simulink model "Controller"  (R2015a)
settings: Solver=ode3  SolverMode=SingleTasking  StartTime=0.0  StopTime=100  FixedStep=T_sim  RelTol=1e-3
PreLoadFcn:
  | LoadLibraries
values from neighbouring files (symbols this model uses):
  a = 10.26    [SetupComplete.m]
  A_x = 0.015    [SetupComplete.m]
  A_y = A_x    (= 0.015)    [SetupComplete.m]
  A_z = 0.16    [SetupComplete.m]
  C_d0 = 0.001193    [SetupComplete.m]
  C_x = 1.2    [SetupComplete.m]
  C_y = C_x    (= 1.2)    [SetupComplete.m]
  C_z = 2.2    [SetupComplete.m]
  CG_0 = [0,0,0.02]'    [SetupComplete.m]
  eta_23 = deg2rad(-1.42)    [Run3Copter.m]
  g = 9.81    [SetupComplete.m]
  h = 0.08    [SetupComplete.m]
  h_M = 0.064    [SetupComplete.m]
  I_BAC_0 = [ Ix,0,Ixz;0,Iy,0;Ixz,0,Iz]    [SetupComplete.m]
  Initial_Omegas = [1;1;1]*Omega_hover    [Run3Copter.m]
  l = 0.3450    (= 0.345)    [NDI_components.m]    (also in SetupComplete.m; robust_controller.m)
  l_arm = 0.264    [SetupComplete.m]
  m = 3.51    [SetupComplete.m]
  m_0 = 2.61    [SetupComplete.m]
  m_M = 0.300    (= 0.3)    [SetupComplete.m]
  R = 0.1778    [SetupComplete.m]    (also in robust_controller.m = eye(4))
  rho = 1.15    [SetupComplete.m]
  sigma = b*c/(pi*R)    (= 0.107416159567)    [SetupComplete.m]
  theta_0 = 0.38397    [SetupComplete.m]
  theta_1 = -0.2967    [SetupComplete.m]
  v_i0 = sqrt( 1/3*m*g/(2*rho*pi*R^2)  )    [SetupComplete.m]
undefined symbols (not defined in the file or in its folder): DOWN_0, EAST_0, Motor, NORTH_0, P_0, Prop, Q_0, R_0, Throttle_Hover, U_0, V_0, v_i_adim, Vx_adim, Vz_adim, W_0
undefined symbols (not defined in the file): Initial_Torques, J_FA, J_T, Rotation_sign, Tau_motors
libraries: XXCopter x39, simulink x35, vrlib x15, simulink_extras x7, aerolib6dofsys x2, qcatlib x2, dspinverses x2
(part 10 of 10)

== matlab function Controller/P Controller/NDI+CA Controller/4DOF NDI+CA Controller/F(X) ==
  data: fx output; prev_input input
function fx = fx(prev_input)
    % Calculates f_hat(x). The expression is calculated in NDI_components
    % x_dot = f(x) + g(x,u)
    %   g(x,u) ~= g(x,u0) + jac(g(x,u), u)(u0) * (u - u0)
    %   g(x,u) ~= h(x,u0) + jac(g(x,u), u)(u0) * u
    % x_dot = f_hat(x) + jac(g(x,u), u) * u
    %   f_hat(x) = f(x) + g(x,u0) - jac(g(x,u), u)(u0) *  u0
    %   g_hat(x) = jac(g(x,u), u)(u0)
    % x_dot = f_hat(x) + g_hat(x) * u
    Ixx = I_BAC(1,1);
    Iyy = I_BAC(2,2);
    Izz = I_BAC(3,3);
    Ixz = I_BAC(1,3);
    Iyz = I_BAC(2,3);
    cx = CG(1);
    cy = CG(2);
    cz = CG(3);
    tau1_0 = prev_input(1);
    eta1_0 = prev_input(2);
    gamma1_0 = prev_input(3);
    tau2_0 = prev_input(4);
    eta2_0 = prev_input(5);
    gamma2_0 = prev_input(6);
    tau3_0 = prev_input(7);
    eta3_0 = prev_input(8);
    gamma3_0 = prev_input(9);

    % TODO Precompute sines and cosines to improve performance. Some
    % repeated terms can also be precomputed
 fx = [...
               (88.941*(6.6073e-7*mass*P^2 + 0.000032054*mass*P*R - 6.6073e-7*mass*R^2 + 0.011243*V*mass*R + 0.011243*Gx - 0.011243*Q*W*mass - 5.7814e-6*eta1_0*mass*tau1_0*cos(eta1_0)))/mass;
 (88.941*(0.011243*Gy - 0.16865*eta1_0*tau1_0*cos(eta1_0) + 7.3537e-7*P*Q*mass + 0.00003163*Q*R*mass + 0.011243*P*W*mass - 0.011243*R*U*mass - 1.7153e-7*eta1_0*mass*tau1_0*sin(eta1_0)))/mass;
                                        -(88.941*(0.000016865*mass*P^2 + 0.011243*V*mass*P + 0.000016865*mass*Q^2 - 0.011243*U*mass*Q - 0.011243*Gz + 0.16865*eta1_0*tau1_0*sin(eta1_0)))/mass;
                                                                                                                               0.010171*eta1_0*tau1_0*sin(eta1_0) - 0.87546*Q*R - 0.043603*P*Q;
                                                                                                                  0.039177*P^2 + 0.90059*P*R - 0.039177*R^2 - 0.3428*eta1_0*tau1_0*cos(eta1_0);
                                                                                                                                0.043603*Q*R - 0.12686*P*Q - 0.20367*eta1_0*tau1_0*sin(eta1_0)];

== matlab function Controller/P Controller/NDI+CA Controller/4DOF NDI+CA Controller - No massic update/F(X) ==
  data: fx output size=[4,1]; prev_input input size=[9,1]; gforce_body input size=[3,1]; omega_body input size=[3,1]; v_body input size=[3,1]
function fx = fx(prev_input, gforce_body, omega_body, v_body)
    % Calculates f_hat(x). The expression is calculated in NDI_components
    % x_dot = f(x) + g(x,u)
    %   g(x,u) ~= g(x,u0) + jac(g(x,u), u)(u0) * (u - u0)
    %   g(x,u) ~= h(x,u0) + jac(g(x,u), u)(u0) * u
    % x_dot = f_hat(x) + jac(g(x,u), u) * u
    %   f_hat(x) = f(x) + g(x,u0) - jac(g(x,u), u)(u0) *  u0
    %   g_hat(x) = jac(g(x,u), u)(u0)
    % x_dot = f_hat(x) + g_hat(x) * u
    tau1_0 = prev_input(1);
    eta1_0 = prev_input(2);
    gamma1_0 = prev_input(3);
    tau2_0 = prev_input(4);
    eta2_0 = prev_input(5);
    gamma2_0 = prev_input(6);
    tau3_0 = prev_input(7);
    eta3_0 = prev_input(8);
    gamma3_0 = prev_input(9);
    Gx =  gforce_body(1);
    Gy =  gforce_body(2);
    Gz =  gforce_body(3);
    U = v_body(1);
    V = v_body(2);
    W = v_body(3);
    P = omega_body(1);
    Q = omega_body(2);
    R = omega_body(3);

    % This matrix was precomputed in NDI_components.m
    % TODO Precompute sines and cosines to improve performance. Some
    % repeated terms can also be precomputed
    
 fx = [... 
                         - 0.0015*P^2 - 1.0*V*P - 0.0015*Q^2 + 1.0*U*Q + 0.2849*Gz - 4.2735*eta1_0*tau1_0*sin(eta1_0);
                  0.89255*eta1_0*tau1_0*cos(eta1_0) - 0.87555*Q*R - 0.043605*P*Q + 0.010171*eta1_0*tau1_0*sin(eta1_0);
     0.039179*P^2 + 0.90066*P*R - 0.039179*R^2 - 0.34281*eta1_0*tau1_0*cos(eta1_0) + 25.344*eta1_0*tau1_0*sin(eta1_0);
                     0.043605*Q*R - 0.12686*P*Q - 15.06*eta1_0*tau1_0*cos(eta1_0) - 0.20367*eta1_0*tau1_0*sin(eta1_0)];

== matlab function Controller/P Controller/NDI+CA Controller/4DOF NDI+CA Controller - No massic update/G(X) 4DOF_WPQR ==
  data: gx output size=[4,4]; prev_input input size=[9,1]
function gx = gx(prev_input)
    % Calculates f_hat(x). The expression is calculated in NDI_components
    % x_dot = f(x) + g(x,u)
    %   g(x,u) ~= g(x,u0) + jac(g(x,u), u)(u0) * (u - u0)
    %   g(x,u) ~= h(x,u0) + jac(g(x,u), u)(u0) * u
    % x_dot = f_hat(x) + jac(g(x,u), u) * u
    %   f_hat(x) = f(x) + g(x,u0) - jac(g(x,u), u)(u0) *  u0
    %   g_hat(x) = jac(g(x,u), u)(u0)
    % x_dot = f_hat(x) + g_hat(x) * u
    tau1_0 = prev_input(1);
    eta1_0 = prev_input(2);
    gamma1_0 = prev_input(3);
    tau2_0 = prev_input(4);
    eta2_0 = prev_input(5);
    gamma2_0 = prev_input(6);
    tau3_0 = prev_input(7);
    eta3_0 = prev_input(8);
    gamma3_0 = prev_input(9);
    
    % This matrix was precomputed in NDI_components.m
    % TODO Precompute sines and cosines to improve performance. Some
    % repeated terms can also be precomputed
    gx = [...
                       -4.274*cos(eta1_0),                                 4.274*tau1_0*sin(eta1_0), -4.274,  -4.274;
 0.01017*cos(eta1_0) - 0.8926*sin(eta1_0), - 0.8926*tau1_0*cos(eta1_0) - 0.01017*tau1_0*sin(eta1_0), -28.02,    28.0;
   25.34*cos(eta1_0) + 0.3428*sin(eta1_0),     0.3428*tau1_0*cos(eta1_0) - 25.34*tau1_0*sin(eta1_0), -12.67,  -12.67;
   15.06*sin(eta1_0) - 0.2037*cos(eta1_0),     15.06*tau1_0*cos(eta1_0) + 0.2037*tau1_0*sin(eta1_0), 0.8549, -0.4475];


 
    
    
    
    
%  0.038016*cos(eta1_0) + 0.00051422*sin(eta1_0), 0.00051422*tau1_0*cos(eta1_0) - 0.038016*tau1_0*sin(eta1_0),    -4.2737*tau1_0, -0.019008,    -4.2737*tau2_0, -0.00051422*tau2_0, -0.019008,   -4.2737*tau3_0, -0.00051422*tau3_0;
%   4.2748*sin(eta1_0) - 0.000015257*cos(eta1_0),  4.2748*tau1_0*cos(eta1_0) + 0.000015257*tau1_0*sin(eta1_0), 0.00065622*tau1_0,  0.042029, 0.00032056*tau2_0,      4.2732*tau2_0, -0.041999, -0.001633*tau3_0,      4.2732*tau3_0;
%                            -4.2735*cos(eta1_0),                                   4.2735*tau1_0*sin(eta1_0),                 0,   -4.2735,                 0,                  0,   -4.2735,                0,                  0;
%     0.010171*cos(eta1_0) - 0.89255*sin(eta1_0),  - 0.89255*tau1_0*cos(eta1_0) - 0.010171*tau1_0*sin(eta1_0),   -0.43748*tau1_0,    -28.02,   -0.21371*tau2_0,     0.23535*tau2_0,    27.999,    1.0887*tau3_0,     0.23535*tau3_0;
%       25.344*cos(eta1_0) + 0.34281*sin(eta1_0),      0.34281*tau1_0*cos(eta1_0) - 25.344*tau1_0*sin(eta1_0),   -0.11019*tau1_0,   -12.672,   -0.11019*tau2_0,    -0.34281*tau2_0,   -12.672,  -0.11019*tau3_0,    -0.34281*tau3_0;
%        15.06*sin(eta1_0) - 0.20367*cos(eta1_0),       15.06*tau1_0*cos(eta1_0) + 0.20367*tau1_0*sin(eta1_0),   0.010171*tau1_0,   0.85486,     13.029*tau2_0,     -7.5251*tau2_0,  -0.44753,    -13.05*tau3_0,     -7.5251*tau3_0];

== matlab function Controller/P Controller/NDI+CA Controller/ 9DOF NDI+CA Controller - No massic update/F(X) 9DOF_UVWPQR ==
  data: fx output size=[6,1]; prev_input input size=[9,1]; gforce_body input size=[3,1]; omega_body input size=[3,1]; v_body input size=[3,1]
function fx = fx(prev_input, gforce_body, omega_body, v_body)
    % Calculates f_hat(x). The expression is calculated in NDI_components
    % x_dot = f(x) + g(x,u)
    %   g(x,u) ~= g(x,u0) + jac(g(x,u), u)(u0) * (u - u0)
    %   g(x,u) ~= h(x,u0) + jac(g(x,u), u)(u0) * u
    % x_dot = f_hat(x) + jac(g(x,u), u) * u
    %   f_hat(x) = f(x) + g(x,u0) - jac(g(x,u), u)(u0) *  u0
    %   g_hat(x) = jac(g(x,u), u)(u0)
    % x_dot = f_hat(x) + g_hat(x) * u
    tau1_0 = prev_input(1);
    eta1_0 = prev_input(2);
    gamma1_0 = prev_input(3);
    tau2_0 = prev_input(4);
    eta2_0 = prev_input(5);
    gamma2_0 = prev_input(6);
    tau3_0 = prev_input(7);
    eta3_0 = prev_input(8);
    gamma3_0 = prev_input(9);
    Gx =  gforce_body(1);
    Gy =  gforce_body(2);
    Gz =  gforce_body(3);
    U = v_body(1);
    V = v_body(2);
    W = v_body(3);
    P = omega_body(1);
    Q = omega_body(2);
    R = omega_body(3);

    % This matrix was precomputed in NDI_components.m
    % TODO Precompute sines and cosines to improve performance. Some
    % repeated terms can also be precomputed
    
 fx = [...
 5.88e-5*P^2 + 0.00285*P*R - 5.88e-5*R^2 + 1.0*V*R + 0.285*Gx - 1.0*Q*W + 4.27*gamma1_0*tau1_0*cos(gamma1_0) + 5.14e-4*gamma2_0*tau2_0*cos(gamma2_0) + 5.14e-4*gamma3_0*tau3_0*cos(gamma3_0) - 5.14e-4*eta1_0*tau1_0*cos(eta1_0)*cos(gamma1_0) + 4.27*eta2_0*tau2_0*cos(eta2_0)*cos(gamma2_0) + 4.27*eta3_0*tau3_0*cos(eta3_0)*cos(gamma3_0) + 0.038*eta1_0*tau1_0*cos(gamma1_0)*sin(eta1_0) - 0.019*eta2_0*tau2_0*cos(gamma2_0)*sin(eta2_0) - 0.019*eta3_0*tau3_0*cos(gamma3_0)*sin(eta3_0) + 0.038*gamma1_0*tau1_0*cos(eta1_0)*sin(gamma1_0) - 0.019*gamma2_0*tau2_0*cos(eta2_0)*sin(gamma2_0) - 0.019*gamma3_0*tau3_0*cos(eta3_0)*sin(gamma3_0) + 5.14e-4*gamma1_0*tau1_0*sin(eta1_0)*sin(gamma1_0) - 4.27*gamma2_0*tau2_0*sin(eta2_0)*sin(gamma2_0) - 4.27*gamma3_0*tau3_0*sin(eta3_0)*sin(gamma3_0);
        0.285*Gy + 6.54e-5*P*Q + 0.00281*Q*R + 1.0*P*W - 1.0*R*U - 6.56e-4*gamma1_0*tau1_0*cos(gamma1_0) - 4.27*gamma2_0*tau2_0*cos(gamma2_0) - 4.27*gamma3_0*tau3_0*cos(gamma3_0) - 4.27*eta1_0*tau1_0*cos(eta1_0)*cos(gamma1_0) - 3.21e-4*eta2_0*tau2_0*cos(eta2_0)*cos(gamma2_0) + 0.00163*eta3_0*tau3_0*cos(eta3_0)*cos(gamma3_0) - 1.53e-5*eta1_0*tau1_0*cos(gamma1_0)*sin(eta1_0) + 0.042*eta2_0*tau2_0*cos(gamma2_0)*sin(eta2_0) - 0.042*eta3_0*tau3_0*cos(gamma3_0)*sin(eta3_0) - 1.53e-5*gamma1_0*tau1_0*cos(eta1_0)*sin(gamma1_0) + 0.042*gamma2_0*tau2_0*cos(eta2_0)*sin(gamma2_0) - 0.042*gamma3_0*tau3_0*cos(eta3_0)*sin(gamma3_0) + 4.27*gamma1_0*tau1_0*sin(eta1_0)*sin(gamma1_0) + 3.21e-4*gamma2_0*tau2_0*sin(eta2_0)*sin(gamma2_0) - 0.00163*gamma3_0*tau3_0*sin(eta3_0)*sin(gamma3_0);
                                                                                                                                                                                                                                                                                                                                                                                                                                                - 0.0015*P^2 - 1.0*V*P - 0.0015*Q^2 + 1.0*U*Q + 0.285*Gz - 4.27*eta1_0*tau1_0*cos(gamma1_0)*sin(eta1_0) - 4.27*eta2_0*tau2_0*cos(gamma2_0)*sin(eta2_0) - 4.27*eta3_0*tau3_0*cos(gamma3_0)*sin(eta3_0) - 4.27*gamma1_0*tau1_0*cos(eta1_0)*sin(gamma1_0) - 4.27*gamma2_0*tau2_0*cos(eta2_0)*sin(gamma2_0) - 4.27*gamma3_0*tau3_0*cos(eta3_0)*sin(gamma3_0);
                                                        0.437*gamma1_0*tau1_0*cos(gamma1_0) - 0.876*Q*R - 0.0436*P*Q - 0.235*gamma2_0*tau2_0*cos(gamma2_0) - 0.235*gamma3_0*tau3_0*cos(gamma3_0) + 0.893*eta1_0*tau1_0*cos(eta1_0)*cos(gamma1_0) + 0.214*eta2_0*tau2_0*cos(eta2_0)*cos(gamma2_0) - 1.09*eta3_0*tau3_0*cos(eta3_0)*cos(gamma3_0) + 0.0102*eta1_0*tau1_0*cos(gamma1_0)*sin(eta1_0) - 28.0*eta2_0*tau2_0*cos(gamma2_0)*sin(eta2_0) + 28.0*eta3_0*tau3_0*cos(gamma3_0)*sin(eta3_0) + 0.0102*gamma1_0*tau1_0*cos(eta1_0)*sin(gamma1_0) - 28.0*gamma2_0*tau2_0*cos(eta2_0)*sin(gamma2_0) + 28.0*gamma3_0*tau3_0*cos(eta3_0)*sin(gamma3_0) - 0.893*gamma1_0*tau1_0*sin(eta1_0)*sin(gamma1_0) - 0.214*gamma2_0*tau2_0*sin(eta2_0)*sin(gamma2_0) + 1.09*gamma3_0*tau3_0*sin(eta3_0)*sin(gamma3_0);
                                                  0.0392*P^2 + 0.901*P*R - 0.0392*R^2 + 0.11*gamma1_0*tau1_0*cos(gamma1_0) + 0.343*gamma2_0*tau2_0*cos(gamma2_0) + 0.343*gamma3_0*tau3_0*cos(gamma3_0) - 0.343*eta1_0*tau1_0*cos(eta1_0)*cos(gamma1_0) + 0.11*eta2_0*tau2_0*cos(eta2_0)*cos(gamma2_0) + 0.11*eta3_0*tau3_0*cos(eta3_0)*cos(gamma3_0) + 25.3*eta1_0*tau1_0*cos(gamma1_0)*sin(eta1_0) - 12.7*eta2_0*tau2_0*cos(gamma2_0)*sin(eta2_0) - 12.7*eta3_0*tau3_0*cos(gamma3_0)*sin(eta3_0) + 25.3*gamma1_0*tau1_0*cos(eta1_0)*sin(gamma1_0) - 12.7*gamma2_0*tau2_0*cos(eta2_0)*sin(gamma2_0) - 12.7*gamma3_0*tau3_0*cos(eta3_0)*sin(gamma3_0) + 0.343*gamma1_0*tau1_0*sin(eta1_0)*sin(gamma1_0) - 0.11*gamma2_0*tau2_0*sin(eta2_0)*sin(gamma2_0) - 0.11*gamma3_0*tau3_0*sin(eta3_0)*sin(gamma3_0);
                                                           0.0436*Q*R - 0.127*P*Q - 0.0102*gamma1_0*tau1_0*cos(gamma1_0) + 7.53*gamma2_0*tau2_0*cos(gamma2_0) + 7.53*gamma3_0*tau3_0*cos(gamma3_0) - 15.1*eta1_0*tau1_0*cos(eta1_0)*cos(gamma1_0) - 13.0*eta2_0*tau2_0*cos(eta2_0)*cos(gamma2_0) + 13.0*eta3_0*tau3_0*cos(eta3_0)*cos(gamma3_0) - 0.204*eta1_0*tau1_0*cos(gamma1_0)*sin(eta1_0) + 0.855*eta2_0*tau2_0*cos(gamma2_0)*sin(eta2_0) - 0.448*eta3_0*tau3_0*cos(gamma3_0)*sin(eta3_0) - 0.204*gamma1_0*tau1_0*cos(eta1_0)*sin(gamma1_0) + 0.855*gamma2_0*tau2_0*cos(eta2_0)*sin(gamma2_0) - 0.448*gamma3_0*tau3_0*cos(eta3_0)*sin(gamma3_0) + 15.1*gamma1_0*tau1_0*sin(eta1_0)*sin(gamma1_0) + 13.0*gamma2_0*tau2_0*sin(eta2_0)*sin(gamma2_0) - 13.0*gamma3_0*tau3_0*sin(eta3_0)*sin(gamma3_0)];

== matlab function Controller/P Controller/NDI+CA Controller/ 9DOF NDI+CA Controller - No massic update/G(X) 9DOF_UVWPQR ==
  data: gx output size=[6,9]; prev_input input size=[9,1]
function gx = gx(prev_input)
    % Calculates f_hat(x). The expression is calculated in NDI_components
    % x_dot = f(x) + g(x,u)
    %   g(x,u) ~= g(x,u0) + jac(g(x,u), u)(u0) * (u - u0)
    %   g(x,u) ~= h(x,u0) + jac(g(x,u), u)(u0) * u
    % x_dot = f_hat(x) + jac(g(x,u), u) * u
    %   f_hat(x) = f(x) + g(x,u0) - jac(g(x,u), u)(u0) *  u0
    %   g_hat(x) = jac(g(x,u), u)(u0)
    % x_dot = f_hat(x) + g_hat(x) * u
    tau1_0 = prev_input(1);
    eta1_0 = prev_input(2);
    gamma1_0 = prev_input(3);
    tau2_0 = prev_input(4);
    eta2_0 = prev_input(5);
    gamma2_0 = prev_input(6);
    tau3_0 = prev_input(7);
    eta3_0 = prev_input(8);
    gamma3_0 = prev_input(9);
    
    % This matrix was precomputed in NDI_components.m
    % TODO Precompute sines and cosines to improve performance. Some
    % repeated terms can also be precomputed
    gx = [...
   5.14e-4*cos(gamma1_0)*sin(eta1_0) - 4.27*sin(gamma1_0) + 0.038*cos(eta1_0)*cos(gamma1_0),  5.14e-4*tau1_0*cos(eta1_0)*cos(gamma1_0) - 0.038*tau1_0*cos(gamma1_0)*sin(eta1_0), - 4.27*tau1_0*cos(gamma1_0) - 0.038*tau1_0*cos(eta1_0)*sin(gamma1_0) - 5.14e-4*tau1_0*sin(eta1_0)*sin(gamma1_0), - 5.14e-4*sin(gamma2_0) - 4.27*cos(gamma2_0)*sin(eta2_0) - 0.019*cos(eta2_0)*cos(gamma2_0),    0.019*tau2_0*cos(gamma2_0)*sin(eta2_0) - 4.27*tau2_0*cos(eta2_0)*cos(gamma2_0), 0.019*tau2_0*cos(eta2_0)*sin(gamma2_0) - 5.14e-4*tau2_0*cos(gamma2_0) + 4.27*tau2_0*sin(eta2_0)*sin(gamma2_0), - 5.14e-4*sin(gamma3_0) - 4.27*cos(gamma3_0)*sin(eta3_0) - 0.019*cos(eta3_0)*cos(gamma3_0),    0.019*tau3_0*cos(gamma3_0)*sin(eta3_0) - 4.27*tau3_0*cos(eta3_0)*cos(gamma3_0), 0.019*tau3_0*cos(eta3_0)*sin(gamma3_0) - 5.14e-4*tau3_0*cos(gamma3_0) + 4.27*tau3_0*sin(eta3_0)*sin(gamma3_0);
 6.56e-4*sin(gamma1_0) + 4.27*cos(gamma1_0)*sin(eta1_0) - 1.53e-5*cos(eta1_0)*cos(gamma1_0),   4.27*tau1_0*cos(eta1_0)*cos(gamma1_0) + 1.53e-5*tau1_0*cos(gamma1_0)*sin(eta1_0), 6.56e-4*tau1_0*cos(gamma1_0) + 1.53e-5*tau1_0*cos(eta1_0)*sin(gamma1_0) - 4.27*tau1_0*sin(eta1_0)*sin(gamma1_0),   4.27*sin(gamma2_0) + 3.21e-4*cos(gamma2_0)*sin(eta2_0) + 0.042*cos(eta2_0)*cos(gamma2_0), 3.21e-4*tau2_0*cos(eta2_0)*cos(gamma2_0) - 0.042*tau2_0*cos(gamma2_0)*sin(eta2_0), 4.27*tau2_0*cos(gamma2_0) - 0.042*tau2_0*cos(eta2_0)*sin(gamma2_0) - 3.21e-4*tau2_0*sin(eta2_0)*sin(gamma2_0),   4.27*sin(gamma3_0) - 0.00163*cos(gamma3_0)*sin(eta3_0) - 0.042*cos(eta3_0)*cos(gamma3_0), 0.042*tau3_0*cos(gamma3_0)*sin(eta3_0) - 0.00163*tau3_0*cos(eta3_0)*cos(gamma3_0), 4.27*tau3_0*cos(gamma3_0) + 0.042*tau3_0*cos(eta3_0)*sin(gamma3_0) + 0.00163*tau3_0*sin(eta3_0)*sin(gamma3_0);
                                                            -4.27*cos(eta1_0)*cos(gamma1_0),                                              4.27*tau1_0*cos(gamma1_0)*sin(eta1_0),                                                                           4.27*tau1_0*cos(eta1_0)*sin(gamma1_0),                                                            -4.27*cos(eta2_0)*cos(gamma2_0),                                             4.27*tau2_0*cos(gamma2_0)*sin(eta2_0),                                                                         4.27*tau2_0*cos(eta2_0)*sin(gamma2_0),                                                            -4.27*cos(eta3_0)*cos(gamma3_0),                                             4.27*tau3_0*cos(gamma3_0)*sin(eta3_0),                                                                         4.27*tau3_0*cos(eta3_0)*sin(gamma3_0);
   0.0102*cos(eta1_0)*cos(gamma1_0) - 0.893*cos(gamma1_0)*sin(eta1_0) - 0.437*sin(gamma1_0), - 0.893*tau1_0*cos(eta1_0)*cos(gamma1_0) - 0.0102*tau1_0*cos(gamma1_0)*sin(eta1_0),   0.893*tau1_0*sin(eta1_0)*sin(gamma1_0) - 0.0102*tau1_0*cos(eta1_0)*sin(gamma1_0) - 0.437*tau1_0*cos(gamma1_0),     0.235*sin(gamma2_0) - 0.214*cos(gamma2_0)*sin(eta2_0) - 28.0*cos(eta2_0)*cos(gamma2_0),    28.0*tau2_0*cos(gamma2_0)*sin(eta2_0) - 0.214*tau2_0*cos(eta2_0)*cos(gamma2_0),   0.235*tau2_0*cos(gamma2_0) + 28.0*tau2_0*cos(eta2_0)*sin(gamma2_0) + 0.214*tau2_0*sin(eta2_0)*sin(gamma2_0),      0.235*sin(gamma3_0) + 1.09*cos(gamma3_0)*sin(eta3_0) + 28.0*cos(eta3_0)*cos(gamma3_0),     1.09*tau3_0*cos(eta3_0)*cos(gamma3_0) - 28.0*tau3_0*cos(gamma3_0)*sin(eta3_0),    0.235*tau3_0*cos(gamma3_0) - 28.0*tau3_0*cos(eta3_0)*sin(gamma3_0) - 1.09*tau3_0*sin(eta3_0)*sin(gamma3_0);
      0.343*cos(gamma1_0)*sin(eta1_0) - 0.11*sin(gamma1_0) + 25.3*cos(eta1_0)*cos(gamma1_0),     0.343*tau1_0*cos(eta1_0)*cos(gamma1_0) - 25.3*tau1_0*cos(gamma1_0)*sin(eta1_0),    - 0.11*tau1_0*cos(gamma1_0) - 25.3*tau1_0*cos(eta1_0)*sin(gamma1_0) - 0.343*tau1_0*sin(eta1_0)*sin(gamma1_0),    - 0.343*sin(gamma2_0) - 0.11*cos(gamma2_0)*sin(eta2_0) - 12.7*cos(eta2_0)*cos(gamma2_0),     12.7*tau2_0*cos(gamma2_0)*sin(eta2_0) - 0.11*tau2_0*cos(eta2_0)*cos(gamma2_0),    12.7*tau2_0*cos(eta2_0)*sin(gamma2_0) - 0.343*tau2_0*cos(gamma2_0) + 0.11*tau2_0*sin(eta2_0)*sin(gamma2_0),    - 0.343*sin(gamma3_0) - 0.11*cos(gamma3_0)*sin(eta3_0) - 12.7*cos(eta3_0)*cos(gamma3_0),     12.7*tau3_0*cos(gamma3_0)*sin(eta3_0) - 0.11*tau3_0*cos(eta3_0)*cos(gamma3_0),    12.7*tau3_0*cos(eta3_0)*sin(gamma3_0) - 0.343*tau3_0*cos(gamma3_0) + 0.11*tau3_0*sin(eta3_0)*sin(gamma3_0);
    0.0102*sin(gamma1_0) + 15.1*cos(gamma1_0)*sin(eta1_0) - 0.204*cos(eta1_0)*cos(gamma1_0),     15.1*tau1_0*cos(eta1_0)*cos(gamma1_0) + 0.204*tau1_0*cos(gamma1_0)*sin(eta1_0),    0.0102*tau1_0*cos(gamma1_0) + 0.204*tau1_0*cos(eta1_0)*sin(gamma1_0) - 15.1*tau1_0*sin(eta1_0)*sin(gamma1_0),      13.0*cos(gamma2_0)*sin(eta2_0) - 7.53*sin(gamma2_0) + 0.855*cos(eta2_0)*cos(gamma2_0),    13.0*tau2_0*cos(eta2_0)*cos(gamma2_0) - 0.855*tau2_0*cos(gamma2_0)*sin(eta2_0),  - 7.53*tau2_0*cos(gamma2_0) - 0.855*tau2_0*cos(eta2_0)*sin(gamma2_0) - 13.0*tau2_0*sin(eta2_0)*sin(gamma2_0),    - 7.53*sin(gamma3_0) - 13.0*cos(gamma3_0)*sin(eta3_0) - 0.448*cos(eta3_0)*cos(gamma3_0),    0.448*tau3_0*cos(gamma3_0)*sin(eta3_0) - 13.0*tau3_0*cos(eta3_0)*cos(gamma3_0),    0.448*tau3_0*cos(eta3_0)*sin(gamma3_0) - 7.53*tau3_0*cos(gamma3_0) + 13.0*tau3_0*sin(eta3_0)*sin(gamma3_0)];
 
    
    
    
    
%  0.038016*cos(eta1_0) + 0.00051422*sin(eta1_0), 0.00051422*tau1_0*cos(eta1_0) - 0.038016*tau1_0*sin(eta1_0),    -4.2737*tau1_0, -0.019008,    -4.2737*tau2_0, -0.00051422*tau2_0, -0.019008,   -4.2737*tau3_0, -0.00051422*tau3_0;
%   4.2748*sin(eta1_0) - 0.000015257*cos(eta1_0),  4.2748*tau1_0*cos(eta1_0) + 0.000015257*tau1_0*sin(eta1_0), 0.00065622*tau1_0,  0.042029, 0.00032056*tau2_0,      4.2732*tau2_0, -0.041999, -0.001633*tau3_0,      4.2732*tau3_0;
%                            -4.2735*cos(eta1_0),                                   4.2735*tau1_0*sin(eta1_0),                 0,   -4.2735,                 0,                  0,   -4.2735,                0,                  0;
%     0.010171*cos(eta1_0) - 0.89255*sin(eta1_0),  - 0.89255*tau1_0*cos(eta1_0) - 0.010171*tau1_0*sin(eta1_0),   -0.43748*tau1_0,    -28.02,   -0.21371*tau2_0,     0.23535*tau2_0,    27.999,    1.0887*tau3_0,     0.23535*tau3_0;
%       25.344*cos(eta1_0) + 0.34281*sin(eta1_0),      0.34281*tau1_0*cos(eta1_0) - 25.344*tau1_0*sin(eta1_0),   -0.11019*tau1_0,   -12.672,   -0.11019*tau2_0,    -0.34281*tau2_0,   -12.672,  -0.11019*tau3_0,    -0.34281*tau3_0;
%        15.06*sin(eta1_0) - 0.20367*cos(eta1_0),       15.06*tau1_0*cos(eta1_0) + 0.20367*tau1_0*sin(eta1_0),   0.010171*tau1_0,   0.85486,     13.029*tau2_0,     -7.5251*tau2_0,  -0.44753,    -13.05*tau3_0,     -7.5251*tau3_0];

== matlab function Controller/3 Copter Simplified1/6dof Eqs of motion/Accelerometer meas ==
  data: Vb input; omega input; omega_dot input; Ab input; A_s output; r_sens parameter
function A_s  = AcellMeas(Vb,omega,omega_dot,Ab, r_sens)




A_s =  Ab + cross(omega,Vb) + cross(omega, cross(omega,r_sens)) +cross(omega_dot,r_sens)  ;

== matlab function Controller/3 Copter Simplified1/6dof Eqs of motion/Position Eqs ==
  data: A_b output; Vb input; omega input; omega_dot input; Forces input; m input; CG input
function A_b  = PositionEqs(Vb,omega,omega_dot, Forces,m, CG)



 
A_b =  1/m*( Forces ) - cross(omega,Vb) - cross(omega, cross(omega,CG)) -cross(omega_dot,CG)  ;

== matlab function Controller/3 Copter Simplified1/6dof Eqs of motion/Rotational eqs ==
  data: omega_dot output; omega_b input; Moments input; I_BAC input
function omega_dot  = Rotational_Eq(omega_b,Moments, I_BAC)



omega_dot =  I_BAC\( Moments - cross(omega_b,I_BAC*omega_b)  );

== matlab function Controller/3 Copter Simplified1/6dof Eqs of motion/SVFI_to_SVFb ==
  data: X_e input; V_e input; X_e_out output; V_b output; omega_b output; Euler_Ang input; Euler_Ang_Dot input; q output
function [X_e_out,V_b, omega_b ,q]=SVFI_to_SVFb(X_e,V_e, Euler_Ang,Euler_Ang_Dot)

xp=V_e(1);
yp=V_e(2);
zp=V_e(3);

phi=Euler_Ang(1);
theta=Euler_Ang(2);
psi=Euler_Ang(3);
phip=Euler_Ang_Dot(1);
thetap=Euler_Ang_Dot(2);
psip=Euler_Ang_Dot(3);

%%
X_e_out=X_e;

q = QuaternionfromEuler(phi,theta,psi); 



HamOut=HamiltonProduct([q(1);-q(2);-q(3);-q(4)],HamiltonProduct([0;xp;yp;zp],[q(1);q(2);q(3);q(4)]) );% q* . v . q
V_b=HamOut(2:4);

omega_b=[phip-psip*sin(theta)  ;
         thetap*cos(phi)+psip*cos(theta)*sin(phi);
            -thetap*sin(phi)+psip*cos(theta)*cos(phi)  ];% Ya que es solo una operacion aislada utilizaremos la ecuaciones con rel trigonometricas
end
function [q]=QuaternionfromEuler(phi,theta,psi)
% options=optimset('MaxFunEvals',3000);
% q=fsolve(@QUATERNIONEULER,[0.6,0.4,0.5,0.4]); % Hay que acertar con los angulos poniendo diferentes valores iniciales del quaternion
%     function F=QUATERNIONEULER(q)
%         F=[ tan(phi)-(2*q(3)*q(4)-2*q(1)*q(2))/(2*q(1)^2+2*q(4)^2-1)  ;
%             sin(-theta)-2*q(2)*q(4)-2*q(1)*q(3);
%             tan(psi)-(2*q(2)*q(3)-2*q(1)*q(4))/(2*q(1)^2+2*q(2)^2-1);
%             q(1)^2+q(2)^2+q(3)^2+q(4)^2-1];
%     end  % Este algoritmo da q* !!!!!

q=[ cos(psi/2)*cos(theta/2)*cos(phi/2)+ sin(psi/2)*sin(theta/2)*sin(phi/2) ;
      cos(psi/2)*cos(theta/2)*sin(phi/2)- sin(psi/2)*sin(theta/2)*cos(phi/2) ;
       cos(psi/2)*sin(theta/2)*cos(phi/2)+ sin(psi/2)*cos(theta/2)*sin(phi/2)   ;
        sin(psi/2)*cos(theta/2)*cos(phi/2)- cos(psi/2)*sin(theta/2)*sin(phi/2)      ]; % Esto nos da q !!!
end

== matlab function Controller/3 Copter Simplified1/6dof Eqs of motion/SV_F_b_to_SV_FI ==
  data: V_b input; q_dot input; q input; V_e output; euler output; euler_dot output
function [V_e,euler,euler_dot]   = SV_F_b_to_SV_FI(  V_b, q_dot,q)

xp=V_b(1);
yp=V_b(2);
zp=V_b(3);

%% Velocity and position in Earth Frame   q . v . q*

SolProd=HamiltonProduct([q(1);q(2);q(3);q(4)],HamiltonProduct([0;xp;yp;zp],[q(1);-q(2);-q(3);-q(4)]) );
V_e=SolProd(2:4);

%% Actitud en Angulos de Euler y sus derivadas. 
euler=[0,0,0]';
euler(1) = atan2(2*q(3)*q(4)+2*q(1)*q(2),2*q(1)^2+2*q(4)^2-1 ); % phi
euler(2) = -asin( 2*q(2)*q(4)-2*q(1)*q(3) ); %  theta
euler(3) = atan2( 2*q(2)*q(3)+2*q(1)*q(4),2*q(1)^2+2*q(2)^2-1 ); %  psi

euler_dot=[0,0,0]';
euler_dot(1,1) = 2/(1+( (2*q(3)*q(4)+2*q(1)*q(2))/(2*q(1)^2+2*q(4)^2-1)  )^2)*[ -(2*q(1)^2*q(2)+ 4*q(1)*q(3)*q(4)-2*q(2)*q(4)^2+q(2))  ,  q(1)*(2*q(1)^2+2*q(4)^2-1)  ,  q(4)*(2*q(1)^2+2*q(4)^2-1)  ,  -(-2*q(1)^2*q(3) +4*q(1)*q(2)*q(4)+2*q(3)*q(4)^2+q(3) ) ]*q_dot.* 1/(2*q(1)^2+2*q(4)^2-1)^2; % Derivada de phi
euler_dot(2,1) = -2/( sqrt(1-4*(q(2)*q(4)-q(1)*q(3))^2)  )*[-q(3),q(4),-q(1),q(2)]*q_dot;  % Theta prima
euler_dot(3,1) = 2/(1+( (2*q(2)*q(3)+2*q(1)*q(4))/(2*q(1)^2+2*q(2)^2-1)  )^2)*[  -(2*q(1)^2*q(4)+4*q(1)*q(2)*q(3)-2*q(2)^2*q(4)+q(4)  ) , 1/2*(q(3)*(4*q(1)^2-4*q(2)^2-2)-8*q(1)*q(2)*q(4) )  ,  q(2)*(2*q(1)^2+2*q(2)^2-1)  , q(1)*(2*q(1)^2+2*q(2)^2-1) ]*q_dot.*1/(2*q(1)^2+2*q(2)^2-1)^2;  % Psi prima



end

== matlab function Controller/3 Copter Simplified1/6dof Eqs of motion/q_dot/Quaternion_dot ==
  data: omega_b input; q_dot output; q input
function q_dot = Quaternion_dot(omega_b,q)


q_dot = 1/2*HamiltonProduct(q,[0;omega_b]);

== matlab function Controller/3 Copter Simplified1/MATLAB Function ==
  data: input input; Tbody_ext output; Mbody_ext output; Kt input; Kq input; v_body input; omega_body input
function [Tbody_ext, Mbody_ext] = fcn(input, Kt, Kq, v_body, omega_body)
    tau1 = input(1);
    eta1 = input(2);
    gamma1 = input(3);
    tau2 = input(4);
    eta2 = input(5);
    gamma2 = input(6);
    tau3 = input(7);
    eta3 = input(8);
    gamma3= input(9);
    U = v_body(1);
    V = v_body(2);
    W = v_body(3);
    P = omega_body(1);
    Q = omega_body(2);
    R = omega_body(3);

Tbody_ext = [...
           - Kt*tau1*sin(gamma1) - Kt*tau2*cos(gamma2)*sin(eta2) - Kt*tau3*cos(gamma3)*sin(eta3);
                       Kt*tau2*sin(gamma2) + Kt*tau3*sin(gamma3) + Kt*tau1*cos(gamma1)*sin(eta1);
 - Kt*tau1*cos(eta1)*cos(gamma1) - Kt*tau2*cos(eta2)*cos(gamma2) - Kt*tau3*cos(eta3)*cos(gamma3)];
 

Mbody_ext = [...
                                                                                                                  (5382319726372233*Kt*tau3*cos(eta3)*cos(gamma3))/18014398509481984 - (5382319726372233*Kt*tau2*cos(eta2)*cos(gamma2))/18014398509481984 - Kq*tau1*sin(gamma1) + Kq*tau2*cos(gamma2)*sin(eta2) + Kq*tau3*cos(gamma3)*sin(eta3);
                                                                                                                                           (69*Kt*tau1*cos(eta1)*cos(gamma1))/200 - Kq*tau3*sin(gamma3) - Kq*tau2*sin(gamma2) - (69*Kt*tau2*cos(eta2)*cos(gamma2))/400 - (69*Kt*tau3*cos(eta3)*cos(gamma3))/400 + Kq*tau1*cos(gamma1)*sin(eta1);
 Kq*tau2*cos(eta2)*cos(gamma2) - (69*Kt*tau3*sin(gamma3))/400 - Kq*tau1*cos(eta1)*cos(gamma1) - (69*Kt*tau2*sin(gamma2))/400 + Kq*tau3*cos(eta3)*cos(gamma3) + (69*Kt*tau1*cos(gamma1)*sin(eta1))/200 + (5382319726372233*Kt*tau2*cos(gamma2)*sin(eta2))/18014398509481984 - (5382319726372233*Kt*tau3*cos(gamma3)*sin(eta3))/18014398509481984];
